simulink model "DCmotor_PID"  (R2025b)
settings: Solver=FixedStepAuto  StartTime=0.0  StopTime=20  FixedStep=0.002  RelTol=1e-3  EnableMultiTasking=on
undefined symbols (not defined in the file): K, tau
settings Model: ExtModeTrigDuration=10000  Creator=LabRyu  LastModifiedBy=User
settings SolverCC: AlgebraicLoopSolver=TrustRegion  PositivePriorityOrder=on
settings DataIOCC: ReturnWorkspaceOutputs=off
settings DebuggingCC: UnconnectedInputMsg=warning  UnconnectedOutputMsg=warning  UnconnectedLineMsg=warning  ArithmeticOperatorsInVariantConditions=warning
settings ModelReferenceCC: EnableRefExpFcnMdlSchedulingChecks=on
settings SFSimCC: SimUseLocalCustomCode=off  CustomCodeUndefinedFunction=UseInterfaceOnly
settings RTWCC: SystemTargetFile=quarc_win64.tlc  TemplateMakefile=quarc_default_tmf  RTWUseLocalCustomCode=off  GPUComputeCapability=3.5  Description=QUARC Win64 Target
settings CodeAppCC: StateflowObjectComments=on
settings STFCustomTargetCC: SystemTargetFile=quarc_win64.tlc  TargetPreCompLibLocation=C:\PROGRA~3\QUARC\lib\2017a\win64\release  TargetLangStandard=C99 (ISO)  StopOnOverrun=off  Debug=off  DownloadToTarget=on
settings GRTTargetCC: ExtMode=on  ExtModeMexFile=quarc_comm  TargetPreCompLibLocation=C:\PROGRA~3\QUARC\lib\2017a\win64\release  ParMdlRefBuildCompliant=off  CompOptLevelCompliant=off  CombineOutputUpdateFcns=off  MatFileLogging=off  CPPClassGenCompliant=off  GRTInterface=on  UseToolchainInfoCompliant=off

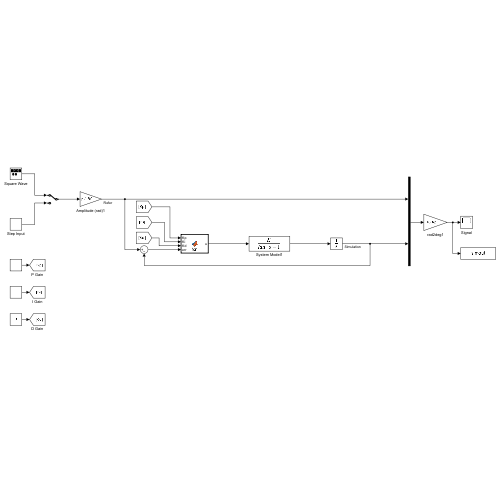
[thumbnail: Simulink's stored preview of the top-level diagram]
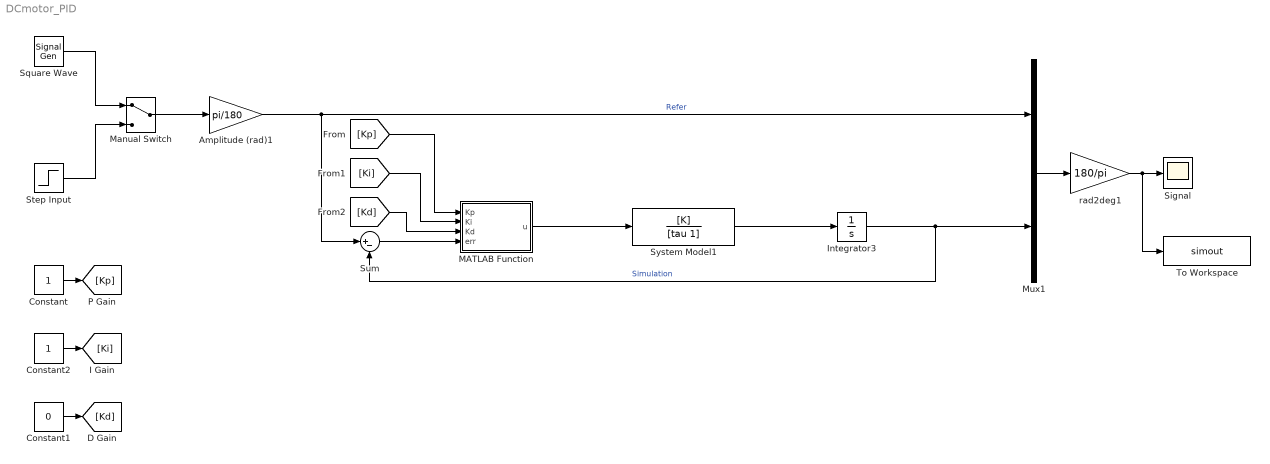
== system DCmotor_PID ==
  Amplitude (rad)1 : Gain  Gain=pi/180
  Constant : Constant
  Constant1 : Constant  Value=0
  Constant2 : Constant
  Integrator3 : Integrator
  MATLAB Function : MATLAB Function  TreatAsAtomicUnit=on
  Manual Switch : ManualSwitch
  Mux1 : Mux  Inputs=2
  Signal : Scope
      settings: TimeSpan=20  ActiveDisplayYMinimum=-88.909851539823222  ActiveDisplayYMaximum=95.171209308998669  DataLoggingMaxPoints=25000  DataLoggingSaveFormat=Array
  Square Wave : SignalGenerator  WaveForm=square  Amplitude=45  Frequency=0.1
  Step Input : Step  SampleTime=0
  Sum : Sum  Inputs=|+-
  System Model1 : TransferFcn  Numerator=[K]  Denominator=[tau 1]
  To Workspace : ToWorkspace  VariableName=simout  SaveFormat=Timeseries  SampleTime=-1
  rad2deg1 : Gain  Gain=180/pi
  wires:
  Mux1/1 -> rad2deg1/1
  rad2deg1/1 -> To Workspace/1, Signal/1
  Amplitude (rad)1/1 -> Sum/1, Mux1/1  "Refer"
  System Model1/1 -> Integrator3/1
  Manual Switch/1 -> Amplitude (rad)1/1
  Square Wave/1 -> Manual Switch/1
  Step Input/1 -> Manual Switch/2
  Constant/1 -> [Kp]
  Sum/1 -> MATLAB Function/4(err)
  [Kp] -> MATLAB Function/1(Kp)
  MATLAB Function/1(u) -> System Model1/1
  Constant1/1 -> [Kd]
  Constant2/1 -> [Ki]
  Integrator3/1 -> Sum/2, Mux1/2  "Simulation"
  [Ki] -> MATLAB Function/2(Ki)
  [Kd] -> MATLAB Function/3(Kd)

== matlab function DCmotor_PID/MATLAB Function ==
  settings: updateMethod=DISCRETE
  data: Kp input; Ki input; Kd input; err input; u output
function u = fcn(Kp, Ki, Kd, err)
    %#codegen
    persistent i_err prev_err dt
    
    if isempty(i_err)
        i_err = 0;
        prev_err = 0;
        dt = 0.001; % or sample time
    end

    i_err = i_err + err * dt;
    d_err = (err - prev_err) / dt;

    u = Kp*err + Ki*i_err + Kd*d_err;

    prev_err = err;
end
